simulink model "foc"  (R2016a)
settings: Solver=VariableStepAuto  StartTime=0.0  StopTime=0.1  MaxStep=1e-4  RelTol=1e-3
settings Model: Creator=ZL  LastModifiedBy=ZL

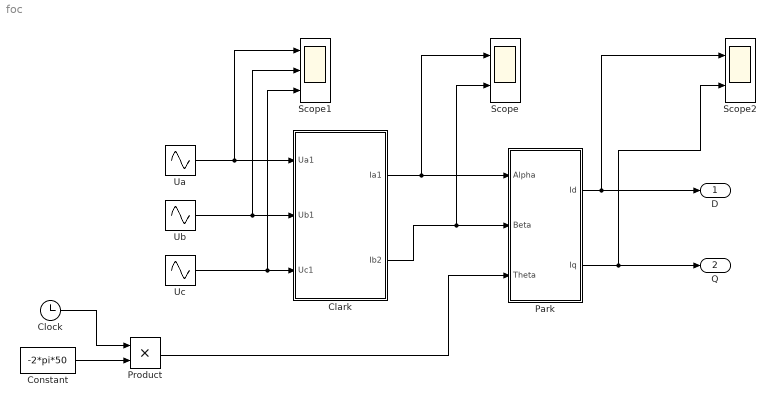
== system foc ==
  " Uc" : Sin  Amplitude=220  Frequency=2*pi*50  Phase=-2*pi/3  SampleTime=0
  Clark : Subsystem
  Clock : Clock
  Constant : Constant  Value=-2*pi*50
  Park : Subsystem
  Product : Product
  Scope : Scope  NumInputPorts=2
  Scope1 : Scope  NumInputPorts=3
  Scope2 : Scope  NumInputPorts=2
  Ua : Sin  Amplitude=220  Frequency=2*pi*50  SampleTime=0
  Ub : Sin  Amplitude=220  Frequency=2*pi*50  Phase=2*pi/3  SampleTime=0
  D : Outport
  Q : Outport  Port=2
  wires:
  Park/1(Id) -> Scope2/1, D/1
  Clark/1(Ia1) -> Scope/1, Park/1(Alpha)
  Clark/2(Ib2) -> Scope/2, Park/2(Beta)
  Constant/1 -> Product/2
  Park/2(Iq) -> Scope2/2, Q/1
  " Uc"/1 -> Scope1/3, Clark/3(Uc1)
  Ub/1 -> Scope1/2, Clark/2(Ub1)
  Ua/1 -> Scope1/1, Clark/1(Ua1)
  Clock/1 -> Product/1
  Product/1 -> Park/3(Theta)

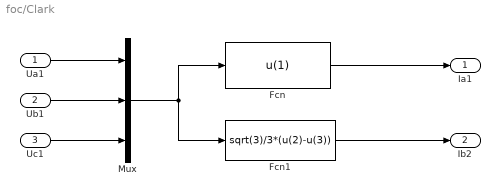
== system foc/Clark ==
  Ua1 : Inport
  Ub1 : Inport  Port=2
  Uc1 : Inport  Port=3
  Fcn : Fcn  Expr=u(1)
  Fcn1 : Fcn  Expr=sqrt(3)/3*(u(2)-u(3))
  Mux : Mux  Inputs=3
  Ia1 : Outport
  Ib2 : Outport  Port=2
  wires:
  Fcn1/1 -> Ib2/1
  Mux/1 -> Fcn/1, Fcn1/1
  Ua1/1 -> Mux/1
  Fcn/1 -> Ia1/1
  Ub1/1 -> Mux/2
  Uc1/1 -> Mux/3

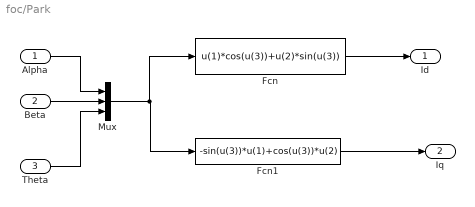
== system foc/Park ==
  Alpha : Inport
  Beta : Inport  Port=2
  Theta : Inport  Port=3
  Fcn : Fcn  Expr=u(1)*cos(u(3))+u(2)*sin(u(3))
  Fcn1 : Fcn  Expr=-sin(u(3))*u(1)+cos(u(3))*u(2)
  Mux : Mux  Inputs=3
  Id : Outport
  Iq : Outport  Port=2
  wires:
  Mux/1 -> Fcn/1, Fcn1/1
  Beta/1 -> Mux/2
  Fcn1/1 -> Iq/1
  Theta/1 -> Mux/3
  Fcn/1 -> Id/1
  Alpha/1 -> Mux/1
